simulink model "untitled"  (Simulink 7.6)
settings: Solver=ode45  StartTime=0.0  StopTime=400.0  RelTol=1e-3
libraries: ADRC x1
settings Model: Creator=Administrator  LastModifiedBy=Administrator
settings DebuggingCC: SolverPrmCheckMsg=none

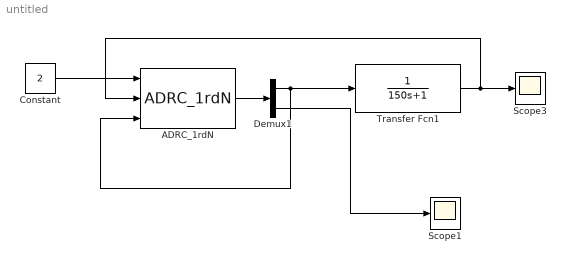
== system untitled ==
  ADRC_1rdN : ADRC/ADRC/ADRC_1rd/ADRC_1rdN  SystemSampleTime=-1  RT=50  h=0.05  B01=20  B02=500  r=1
  Constant : Constant  Value=2
  Demux1 : Demux  Outputs=2
  Scope1 : Scope
      settings: TimeRange=1000  YMin=-2e+235  YMax=1.4e+236  DataFormat=Array
  Scope3 : Scope
      settings: TimeRange=1000  YMin=-2e+235  YMax=1.4e+236  DataFormat=Array
  Transfer Fcn1 : TransferFcn  Numerator=1  Denominator=[150 1]
  wires:
  Constant/1 -> ADRC_1rdN/1
  Transfer Fcn1/1 -> Scope3/1, ADRC_1rdN/2
  ADRC_1rdN/1 -> Demux1/1
  Demux1/1 -> Transfer Fcn1/1, ADRC_1rdN/3
  Demux1/2 -> Scope1/1
